simulink model "sst_cllc_ttype_inv"  (R2026a)
settings: Solver=ode23tb  StopTime=simlength  FixedStep=tc  MaxStep=glb_time.tc
values from neighbouring files (symbols this model uses):
  afe_ctrl = ctrl_afe_setup(glb_time.ts_afe, grid_emu.omega_grid_nom)    [init_model.m]
  cllc_ctrl = ctrl_cllc_setup(kp_udc, ki_udc, kp_idc, ki_idc)    [init_model.m]
  glb_time = timing_setup(fpwm_afe, trgo_afe, fpwm_inv, trgo_inv, fpwm_single_phase_inv, trgo_single_phase_inv, fpwm_dab, trgo_dab,      fpwm_psfbc, trgo_psfbc, fpwm_isop_rail, trgo_isop_rail, fpwm_cllc, trgo_cllc, t_measure, tc_factor, tc_decimation, delay_pwm, dead_time_afe,      dead_time_inv, dead_time_single_phase_inv, dead_time_dab, dead_time_psfbc, dead_time_isop_rail, dead_time_cllc)    [init_model.m]
  grid_emu = grid_three_phase_emulator('Dyn11', delta_star, grid_nominal_power, application_voltage, us1, us2, fgrid,                  eq_grid_inductance, eq_grid_resistance, eta, ucc, i1m, p_iron, n1, n2, core_area, core_length, mur,                  up_xi_pu_ref, up_eta_pu_ref, un_xi_pu_ref, un_eta_pu_ref)    [init_model.m]
  lithium_ion_battery_1 = lithium_ion_battery_setup(nominal_battery_voltage_1, nominal_battery_power, initial_battery_soc, glb_time.ts_dab)    [init_model.m]
  omega_set = frequency_set*2*pi    (= 1884.95559215)    [init_model.m]
  single_phase_inverter_ctrl = ctrl_single_phase_inverter_setup(glb_time.ts_inv, pres_ctrl.omega_set,      dqvector_pi.kp_inv, dqvector_pi.ki_inv, pres_ctrl.kp_rpi, pres_ctrl.ki_rpi, pres_ctrl.delta_rpi)    [init_model.m]
  sst_num_of_modules = 2    [init_model.m]
undefined symbols (not defined in the file or in its folder): hwdata
libraries: fl_lib x62, nesl_utility x38, discrete_time_low_pass_filter x8, full_bridge_ideal_switch x4, full_bridge_mosfet_based_with_thermal_model x4, full_bridge_mosfet_based_with_thermal_model_zvs x4, lithium_ion_battery x2, single_phase_transformer x2, dab_single_phase_pwm_modulator x2, dclink_for_three_levels x2, full_bridge_three_level_ttype_ideal_switch_based_model x2, full_bridge_three_level_ttype_mosfet_based_model x2
(part 4 of 5)

== system sst_cllc_ttype_inv/single_phase_inverter_modA/single phase inverter control/single_phase_inverter_ctrl/scopes ==
  Bus Creator1 : BusCreator  Inputs=3
  Bus Creator2 : BusCreator  Inputs=2
  Bus Creator3 : BusCreator  Inputs=2
  Bus Creator4 : BusCreator  Inputs=2
  single phase inverter tracking current scope 1 : Scope  NumInputPorts=2
      settings: ActiveDisplayYMinimum=-1.23468017578125  ActiveDisplayYMaximum=1.23419189453125  DataLoggingVariableName=ScopeData12
  single phase inverter tracking current scope 2 : Scope  NumInputPorts=2
      settings: ActiveDisplayYMinimum=-1.2603759765625  ActiveDisplayYMaximum=1.2652587890625  DataLoggingVariableName=ScopeData2
  wires:
  Bus Creator1/1 -> single phase inverter tracking current scope 1/2  "is_tracking"
  [i_out_alphabeta_ref] -> Bus Creator1/2  "i_out_inverter_pu_ref"
  [afe_current_output_pu] -> Bus Creator1/3  "inverter_current_output_pu"
  [afe_voltage_output_pu] -> Bus Creator2/1  "inverter_voltage_output_pu"
  Bus Creator2/1 -> single phase inverter tracking current scope 1/1  "load"
  [inverter_current_output_pu_reference] -> Bus Creator1/1  "inverter_current_output_pu_reference"
  [afe_current_output_pu] -> Bus Creator2/2  "inverter_current_output_pu"
  [u_ctrl_out] -> Bus Creator3/1  "u_ctrl_out"
  [afe_voltage_output_pu] -> Bus Creator3/2  "inverter_voltage_output_pu"
  Bus Creator3/1 -> single phase inverter tracking current scope 2/2  "u_load"
  [afe_current_output_pu] -> Bus Creator4/2  "inverter_current_output_pu"
  [i_out_alphabeta_ref] -> Bus Creator4/1  "i_out_alphabeta_ref"
  Bus Creator4/1 -> single phase inverter tracking current scope 2/1  "i_load"

== system sst_cllc_ttype_inv/single_phase_inverter_modA/single phase inverter control/single_phase_inverter_ctrl/single_phase_current_control ==
  inverter_current_output_pu_reference : Inport
  current_reference_generation : Subsystem
  dqpi_current_controller : Subsystem
  u_ctrl_out : Outport
  tag scope: i_out_alphabeta_ref=scoped, inverter_current_output_pu_reference=scoped, u_ctrl_out=scoped
  wires:
  current_reference_generation/1(is_ref) -> [i_out_alphabeta_ref]  "i_out_inverter_pu_ref"
  dqpi_current_controller/1(u_out) -> u_ctrl_out/1, [u_ctrl_out]  "u_ctrl_out"
  [phase_grid] -> current_reference_generation/2(phase)
  inverter_current_output_pu_reference/1 -> current_reference_generation/1(mag_ref), [inverter_current_output_pu_reference]
  current_reference_generation/2(id_ref) -> dqpi_current_controller/1(id_ref)

== system sst_cllc_ttype_inv/single_phase_inverter_modA/single phase inverter control/single_phase_inverter_ctrl/single_phase_pll ==
  input : Inport
  Constant : Constant
  Constant2 : Constant  Value=0
  Scope : Scope  NumInputPorts=2
      settings: ActiveDisplayYMinimum=-3.2854912154015015  ActiveDisplayYMaximum=3.4773424919151528
  Sum : Sum  Inputs=|++
  Sum1 : Sum  Inputs=|++
  Terminator : Terminator
  Terminator1 : Terminator
  Terminator2 : Terminator
  Unit Delay1 : UnitDelay  SampleTime=-1
  alphabeta2xieta : MATLAB Function  TreatAsAtomicUnit=on
  bounder2 : MATLAB Function  TreatAsAtomicUnit=on
  double_integrator_observer : Subsystem
  freq_pll : Gain  Gain=1/2/pi
  omega_int_ts : Gain  Gain=omega_set * glb_time.ts_inv
  pi-ctrl : Subsystem  mask{kp=1, ki=0, ts=glb_time.ts_inv, sat_pos=2, sat_neg=-2}
  ualpha_pll : Gain
  ubeta_pll : Gain
  ueta_pll : Gain  Gain=-1
  ueta_pll_flt : discrete_time_low_pass_filter/discrete-time-low-pass-filter  tau=2/omega_set  ts=glb_time.ts_inv
  uxi_pll : Gain
  uxi_pll_flt : discrete_time_low_pass_filter/discrete-time-low-pass-filter  tau=2/omega_set  ts=glb_time.ts_inv
  xieta2alphabeta : MATLAB Function  TreatAsAtomicUnit=on
  phase_pll_hat : Outport
  omega_pll_hat : Outport  Port=2
  wires:
  Sum/1 -> bounder2/1(u)
  alphabeta2xieta/1(xi) -> uxi_pll/1, uxi_pll_flt/1
  xieta2alphabeta/2(beta) -> ubeta_pll/1
  alphabeta2xieta/2(eta) -> ueta_pll/1, ueta_pll_flt/1
  omega_int_ts/1 -> freq_pll/1, Sum/1
  double_integrator_observer/1(phase_hat) -> Scope/1, phase_pll_hat/1  "phase_pll_hat"
  input/1 -> alphabeta2xieta/1(alpha)
  freq_pll/1 -> Terminator1/1  "freq_pll"
  ueta_pll_flt/1 -> xieta2alphabeta/2(eta)
  uxi_pll_flt/1 -> xieta2alphabeta/1(xi)
  ueta_pll/1 -> pi-ctrl/1(x)
  Sum1/1 -> omega_int_ts/1  "freq_pll"
  Constant2/1 -> pi-ctrl/2(xref)
  uxi_pll/1 -> Terminator2/1
  ubeta_pll/1 -> alphabeta2xieta/2(beta)
  xieta2alphabeta/1(alpha) -> ualpha_pll/1
  pi-ctrl/1(u) -> Sum1/1
  Constant/1 -> Sum1/2
  Unit Delay1/1 -> Sum/2, alphabeta2xieta/3(gamma), xieta2alphabeta/3(gamma), double_integrator_observer/1(theta)
  bounder2/1(y) -> Unit Delay1/1  "theta_hat_bounded"
  double_integrator_observer/2(omega_hat) -> Scope/2, omega_pll_hat/1  "omega_pll_hat"
  ualpha_pll/1 -> Terminator/1

== system sst_cllc_ttype_inv/single_phase_inverter_modA/single phase inverter control/single_phase_inverter_ctrl/storage_data ==
  To Workspace : ToWorkspace  VariableName=inverter_voltage_output_pu_sim  SampleTime=-1
      settings: MaxDataPoints=glb_time.Ns_inv  Save2DSignal=2-D array (concatenate along first dimension)
  To Workspace1 : ToWorkspace  VariableName=inverter_current_output_pu_sim  SampleTime=-1
      settings: MaxDataPoints=glb_time.Ns_inv  Save2DSignal=2-D array (concatenate along first dimension)
  To Workspace10 : ToWorkspace  VariableName=iq_pu_ref_sim  SampleTime=-1
      settings: MaxDataPoints=glb_time.Ns_inv  Save2DSignal=2-D array (concatenate along first dimension)
  To Workspace11 : ToWorkspace  VariableName=iq_pu_sim  SampleTime=-1
      settings: MaxDataPoints=glb_time.Ns_inv  Save2DSignal=2-D array (concatenate along first dimension)
  To Workspace12 : ToWorkspace  VariableName=ud_ctrl_out_sim  SampleTime=-1
      settings: MaxDataPoints=glb_time.Ns_inv  Save2DSignal=2-D array (concatenate along first dimension)
  To Workspace13 : ToWorkspace  VariableName=uq_ctrl_out_sim  SampleTime=-1
      settings: MaxDataPoints=glb_time.Ns_inv  Save2DSignal=2-D array (concatenate along first dimension)
  To Workspace2 : ToWorkspace  VariableName=inverter_current_output_pu_reference_sim  SampleTime=-1
      settings: MaxDataPoints=glb_time.Ns_inv  Save2DSignal=2-D array (concatenate along first dimension)
  To Workspace3 : ToWorkspace  VariableName=i_out_inverter_pu_ref_sim  SampleTime=-1
      settings: MaxDataPoints=glb_time.Ns_inv  Save2DSignal=2-D array (concatenate along first dimension)
  To Workspace4 : ToWorkspace  VariableName=u_ctrl_out_sim  SampleTime=-1
      settings: MaxDataPoints=glb_time.Ns_inv  Save2DSignal=2-D array (concatenate along first dimension)
  To Workspace5 : ToWorkspace  VariableName=time_ts_inv_sim  SampleTime=-1
      settings: MaxDataPoints=glb_time.Ns_inv  Save2DSignal=2-D array (concatenate along first dimension)
  To Workspace6 : ToWorkspace  VariableName=i_alpha_pu_sim  SampleTime=-1
      settings: MaxDataPoints=glb_time.Ns_inv  Save2DSignal=2-D array (concatenate along first dimension)
  To Workspace7 : ToWorkspace  VariableName=i_beta_pu_sim  SampleTime=-1
      settings: MaxDataPoints=glb_time.Ns_inv  Save2DSignal=2-D array (concatenate along first dimension)
  To Workspace8 : ToWorkspace  VariableName=id_pu_ref_sim  SampleTime=-1
      settings: MaxDataPoints=glb_time.Ns_inv  Save2DSignal=2-D array (concatenate along first dimension)
  To Workspace9 : ToWorkspace  VariableName=id_pu_sim  SampleTime=-1
      settings: MaxDataPoints=glb_time.Ns_inv  Save2DSignal=2-D array (concatenate along first dimension)
  wires:
  [afe_voltage_output_pu] -> To Workspace/1  "inverter_voltage_output_pu"
  [afe_current_output_pu] -> To Workspace1/1  "inverter_current_output_pu"
  [inverter_current_output_pu_reference] -> To Workspace2/1  "inverter_current_output_pu_reference"
  [i_out_alphabeta_ref] -> To Workspace3/1  "i_out_inverter_pu_ref"
  [u_ctrl_out] -> To Workspace4/1  "u_ctrl_out"
  [local_time] -> To Workspace5/1
  [i_alpha] -> To Workspace6/1
  [i_beta] -> To Workspace7/1
  [id_ref] -> To Workspace8/1
  [id] -> To Workspace9/1
  [iq_ref] -> To Workspace10/1
  [iq] -> To Workspace11/1
  [ud_ctrl] -> To Workspace12/1
  [uq_ctrl] -> To Workspace13/1

== system sst_cllc_ttype_inv/single_phase_inverter_modB/single phase inverter control/single_phase_inverter_ctrl/scopes ==
  Bus Creator1 : BusCreator  Inputs=3
  Bus Creator2 : BusCreator  Inputs=2
  Bus Creator3 : BusCreator  Inputs=2
  Bus Creator4 : BusCreator  Inputs=2
  single phase inverter tracking current scope 1 : Scope  NumInputPorts=2
      settings: ActiveDisplayYMinimum=-1.23468017578125  ActiveDisplayYMaximum=1.23419189453125  DataLoggingVariableName=ScopeData12
  single phase inverter tracking current scope 2 : Scope  NumInputPorts=2
      settings: ActiveDisplayYMinimum=-1.2603759765625  ActiveDisplayYMaximum=1.2652587890625  DataLoggingVariableName=ScopeData2
  wires:
  Bus Creator4/1 -> single phase inverter tracking current scope 2/1  "i_load"
  [i_out_alphabeta_ref] -> Bus Creator4/1  "i_out_alphabeta_ref"
  [afe_current_output_pu] -> Bus Creator4/2  "inverter_current_output_pu"
  Bus Creator3/1 -> single phase inverter tracking current scope 2/2  "u_load"
  [afe_voltage_output_pu] -> Bus Creator3/2  "inverter_voltage_output_pu"
  [u_ctrl_out] -> Bus Creator3/1  "u_ctrl_out"
  [afe_current_output_pu] -> Bus Creator2/2  "inverter_current_output_pu"
  [inverter_current_output_pu_reference] -> Bus Creator1/1  "inverter_current_output_pu_reference"
  Bus Creator2/1 -> single phase inverter tracking current scope 1/1  "load"
  [afe_voltage_output_pu] -> Bus Creator2/1  "inverter_voltage_output_pu"
  [afe_current_output_pu] -> Bus Creator1/3  "inverter_current_output_pu"
  [i_out_alphabeta_ref] -> Bus Creator1/2  "i_out_inverter_pu_ref"
  Bus Creator1/1 -> single phase inverter tracking current scope 1/2  "is_tracking"

== system sst_cllc_ttype_inv/single_phase_inverter_modB/single phase inverter control/single_phase_inverter_ctrl/single_phase_current_control ==
  inverter_current_output_pu_reference : Inport
  current_reference_generation : Subsystem
  dqpi_current_controller : Subsystem
  u_ctrl_out : Outport
  tag scope: i_out_alphabeta_ref=scoped, inverter_current_output_pu_reference=scoped, u_ctrl_out=scoped
  wires:
  current_reference_generation/2(id_ref) -> dqpi_current_controller/1(id_ref)
  inverter_current_output_pu_reference/1 -> [inverter_current_output_pu_reference], current_reference_generation/1(mag_ref)
  [phase_grid] -> current_reference_generation/2(phase)
  dqpi_current_controller/1(u_out) -> [u_ctrl_out], u_ctrl_out/1  "u_ctrl_out"
  current_reference_generation/1(is_ref) -> [i_out_alphabeta_ref]  "i_out_inverter_pu_ref"

== system sst_cllc_ttype_inv/single_phase_inverter_modB/single phase inverter control/single_phase_inverter_ctrl/single_phase_pll ==
  input : Inport
  Constant : Constant
  Constant2 : Constant  Value=0
  Scope : Scope  NumInputPorts=2
      settings: ActiveDisplayYMinimum=-3.2854912154015015  ActiveDisplayYMaximum=3.4773424919151528
  Sum : Sum  Inputs=|++
  Sum1 : Sum  Inputs=|++
  Terminator : Terminator
  Terminator1 : Terminator
  Terminator2 : Terminator
  Unit Delay1 : UnitDelay  SampleTime=-1
  alphabeta2xieta : MATLAB Function  TreatAsAtomicUnit=on
  bounder2 : MATLAB Function  TreatAsAtomicUnit=on
  double_integrator_observer : Subsystem
  freq_pll : Gain  Gain=1/2/pi
  omega_int_ts : Gain  Gain=omega_set * glb_time.ts_inv
  pi-ctrl : Subsystem  mask{kp=1, ki=0, ts=glb_time.ts_inv, sat_pos=2, sat_neg=-2}
  ualpha_pll : Gain
  ubeta_pll : Gain
  ueta_pll : Gain  Gain=-1
  ueta_pll_flt : discrete_time_low_pass_filter/discrete-time-low-pass-filter  tau=2/omega_set  ts=glb_time.ts_inv
  uxi_pll : Gain
  uxi_pll_flt : discrete_time_low_pass_filter/discrete-time-low-pass-filter  tau=2/omega_set  ts=glb_time.ts_inv
  xieta2alphabeta : MATLAB Function  TreatAsAtomicUnit=on
  phase_pll_hat : Outport
  omega_pll_hat : Outport  Port=2
  wires:
  ualpha_pll/1 -> Terminator/1
  double_integrator_observer/2(omega_hat) -> omega_pll_hat/1, Scope/2  "omega_pll_hat"
  bounder2/1(y) -> Unit Delay1/1  "theta_hat_bounded"
  Unit Delay1/1 -> double_integrator_observer/1(theta), xieta2alphabeta/3(gamma), alphabeta2xieta/3(gamma), Sum/2
  Constant/1 -> Sum1/2
  pi-ctrl/1(u) -> Sum1/1
  xieta2alphabeta/1(alpha) -> ualpha_pll/1
  ubeta_pll/1 -> alphabeta2xieta/2(beta)
  uxi_pll/1 -> Terminator2/1
  Constant2/1 -> pi-ctrl/2(xref)
  Sum1/1 -> omega_int_ts/1  "freq_pll"
  ueta_pll/1 -> pi-ctrl/1(x)
  uxi_pll_flt/1 -> xieta2alphabeta/1(xi)
  ueta_pll_flt/1 -> xieta2alphabeta/2(eta)
  freq_pll/1 -> Terminator1/1  "freq_pll"
  input/1 -> alphabeta2xieta/1(alpha)
  double_integrator_observer/1(phase_hat) -> phase_pll_hat/1, Scope/1  "phase_pll_hat"
  omega_int_ts/1 -> Sum/1, freq_pll/1
  alphabeta2xieta/2(eta) -> ueta_pll_flt/1, ueta_pll/1
  xieta2alphabeta/2(beta) -> ubeta_pll/1
  alphabeta2xieta/1(xi) -> uxi_pll_flt/1, uxi_pll/1
  Sum/1 -> bounder2/1(u)

== system sst_cllc_ttype_inv/single_phase_inverter_modB/single phase inverter control/single_phase_inverter_ctrl/storage_data ==
  To Workspace : ToWorkspace  VariableName=inverter_voltage_output_pu_sim  SampleTime=-1
      settings: MaxDataPoints=glb_time.Ns_inv  Save2DSignal=2-D array (concatenate along first dimension)
  To Workspace1 : ToWorkspace  VariableName=inverter_current_output_pu_sim  SampleTime=-1
      settings: MaxDataPoints=glb_time.Ns_inv  Save2DSignal=2-D array (concatenate along first dimension)
  To Workspace10 : ToWorkspace  VariableName=iq_pu_ref_sim  SampleTime=-1
      settings: MaxDataPoints=glb_time.Ns_inv  Save2DSignal=2-D array (concatenate along first dimension)
  To Workspace11 : ToWorkspace  VariableName=iq_pu_sim  SampleTime=-1
      settings: MaxDataPoints=glb_time.Ns_inv  Save2DSignal=2-D array (concatenate along first dimension)
  To Workspace12 : ToWorkspace  VariableName=ud_ctrl_out_sim  SampleTime=-1
      settings: MaxDataPoints=glb_time.Ns_inv  Save2DSignal=2-D array (concatenate along first dimension)
  To Workspace13 : ToWorkspace  VariableName=uq_ctrl_out_sim  SampleTime=-1
      settings: MaxDataPoints=glb_time.Ns_inv  Save2DSignal=2-D array (concatenate along first dimension)
  To Workspace2 : ToWorkspace  VariableName=inverter_current_output_pu_reference_sim  SampleTime=-1
      settings: MaxDataPoints=glb_time.Ns_inv  Save2DSignal=2-D array (concatenate along first dimension)
  To Workspace3 : ToWorkspace  VariableName=i_out_inverter_pu_ref_sim  SampleTime=-1
      settings: MaxDataPoints=glb_time.Ns_inv  Save2DSignal=2-D array (concatenate along first dimension)
  To Workspace4 : ToWorkspace  VariableName=u_ctrl_out_sim  SampleTime=-1
      settings: MaxDataPoints=glb_time.Ns_inv  Save2DSignal=2-D array (concatenate along first dimension)
  To Workspace5 : ToWorkspace  VariableName=time_ts_inv_sim  SampleTime=-1
      settings: MaxDataPoints=glb_time.Ns_inv  Save2DSignal=2-D array (concatenate along first dimension)
  To Workspace6 : ToWorkspace  VariableName=i_alpha_pu_sim  SampleTime=-1
      settings: MaxDataPoints=glb_time.Ns_inv  Save2DSignal=2-D array (concatenate along first dimension)
  To Workspace7 : ToWorkspace  VariableName=i_beta_pu_sim  SampleTime=-1
      settings: MaxDataPoints=glb_time.Ns_inv  Save2DSignal=2-D array (concatenate along first dimension)
  To Workspace8 : ToWorkspace  VariableName=id_pu_ref_sim  SampleTime=-1
      settings: MaxDataPoints=glb_time.Ns_inv  Save2DSignal=2-D array (concatenate along first dimension)
  To Workspace9 : ToWorkspace  VariableName=id_pu_sim  SampleTime=-1
      settings: MaxDataPoints=glb_time.Ns_inv  Save2DSignal=2-D array (concatenate along first dimension)
  wires:
  [uq_ctrl] -> To Workspace13/1
  [ud_ctrl] -> To Workspace12/1
  [iq] -> To Workspace11/1
  [iq_ref] -> To Workspace10/1
  [id] -> To Workspace9/1
  [id_ref] -> To Workspace8/1
  [i_beta] -> To Workspace7/1
  [i_alpha] -> To Workspace6/1
  [local_time] -> To Workspace5/1
  [u_ctrl_out] -> To Workspace4/1  "u_ctrl_out"
  [i_out_alphabeta_ref] -> To Workspace3/1  "i_out_inverter_pu_ref"
  [inverter_current_output_pu_reference] -> To Workspace2/1  "inverter_current_output_pu_reference"
  [afe_current_output_pu] -> To Workspace1/1  "inverter_current_output_pu"
  [afe_voltage_output_pu] -> To Workspace/1  "inverter_voltage_output_pu"

== system sst_cllc_ttype_inv/dcdc_cllc_modA/dcdc_with_galvanic_isolation/full-bridge_1/full-bridge_ideal_switch_based/data_measure ==
  m : Inport
  Bus Selector1 : BusSelector  OutputSignals=ideal_switch_current_Q2,ideal_switch_voltage_Q2
  Bus Selector2 : BusSelector  OutputSignals=ideal_switch_current_Q1,ideal_switch_voltage_Q1
  tag scope: idevice_ids_cllc_Q1_modA=global, idevice_ids_cllc_Q2_modA=global, idevice_uds_cllc_Q1_modA=global, idevice_uds_cllc_Q2_modA=global
  wires:
  Bus Selector1/1 -> [idevice_ids_cllc_Q2_modA]  "<ideal_switch_current_Q2>"
  Bus Selector1/2 -> [idevice_uds_cllc_Q2_modA]  "<ideal_switch_voltage_Q2>"
  m/1 -> Bus Selector2/1, Bus Selector1/1
  Bus Selector2/1 -> [idevice_ids_cllc_Q1_modA]  "<ideal_switch_current_Q1>"
  Bus Selector2/2 -> [idevice_uds_cllc_Q1_modA]  "<ideal_switch_voltage_Q1>"

== system sst_cllc_ttype_inv/dcdc_cllc_modA/dcdc_with_galvanic_isolation/full-bridge_1/full-bridge_mosfet_based_with_thermal_model/data_measure ==
  m : Inport
  tag scope: inverter_1_cllc_mosfet_modA=global
  wires:
  m/1 -> [inverter_1_cllc_mosfet_modA]

== system sst_cllc_ttype_inv/dcdc_cllc_modA/dcdc_with_galvanic_isolation/full-bridge_1/full-bridge_mosfet_based_with_thermal_model_zvs/data_measure ==
  m : Inport
  tag scope: inverter_1_cllc_mosfet_zvs_modA=global
  wires:
  m/1 -> [inverter_1_cllc_mosfet_zvs_modA]

== system sst_cllc_ttype_inv/dcdc_cllc_modA/dcdc_with_galvanic_isolation/full-bridge_2/full-bridge_ideal_switch_based/data_measure ==
  m : Inport
  Bus Selector1 : BusSelector  OutputSignals=ideal_switch_current_Q2,ideal_switch_voltage_Q2
  Bus Selector2 : BusSelector  OutputSignals=ideal_switch_current_Q1,ideal_switch_voltage_Q1
  tag scope: idevice_ids_cllc_Q5_modA=global, idevice_ids_cllc_Q6_modA=global, idevice_uds_cllc_Q5_modA=global, idevice_uds_cllc_Q6_modA=global
  wires:
  Bus Selector1/1 -> [idevice_ids_cllc_Q6_modA]  "<ideal_switch_current_Q2>"
  Bus Selector1/2 -> [idevice_uds_cllc_Q6_modA]  "<ideal_switch_voltage_Q2>"
  m/1 -> Bus Selector2/1, Bus Selector1/1
  Bus Selector2/1 -> [idevice_ids_cllc_Q5_modA]  "<ideal_switch_current_Q1>"
  Bus Selector2/2 -> [idevice_uds_cllc_Q5_modA]  "<ideal_switch_voltage_Q1>"

== system sst_cllc_ttype_inv/dcdc_cllc_modA/dcdc_with_galvanic_isolation/full-bridge_2/full-bridge_mosfet_based_with_thermal_model/data_measure ==
  m : Inport
  tag scope: inverter_2_cllc_mosfet_modA=global
  wires:
  m/1 -> [inverter_2_cllc_mosfet_modA]

== system sst_cllc_ttype_inv/dcdc_cllc_modA/dcdc_with_galvanic_isolation/full-bridge_2/full-bridge_mosfet_based_with_thermal_model_zvs/data_measure ==
  m : Inport
  tag scope: inverter_2_cllc_mosfet_zvs_modA=global
  wires:
  m/1 -> [inverter_2_cllc_mosfet_zvs_modA]

== system sst_cllc_ttype_inv/dcdc_cllc_modA/input_current_control/input_current_control/inner_ctrl/current_control ==
  i_ref : Inport
  i : Inport  Port=2
  Gain : Gain  Gain=-1
  Sum2 : Sum  Inputs=+-  OutDataTypeStr=double  AccumDataTypeStr=double  SaturateOnIntegerOverflow=on
  Unit Delay2 : UnitDelay  SampleTime=-1
  i_ctrl : Subsystem
  ctrli_out : Outport
  wires:
  i/1 -> Sum2/2
  i_ref/1 -> Sum2/1
  Sum2/1 -> i_ctrl/1(i_tilde)
  Gain/1 -> Unit Delay2/1
  i_ctrl/1(phase_shift) -> Gain/1
  Unit Delay2/1 -> ctrli_out/1  "current_ctrl_output"

== system sst_cllc_ttype_inv/dcdc_cllc_modA/input_current_control/input_current_control/outer_ctrl/current_control ==
  iout_ref : Inport
  iout : Inport  Port=2
  Gain : Gain
  Sum2 : Sum  Inputs=+-  OutDataTypeStr=double  AccumDataTypeStr=double  SaturateOnIntegerOverflow=on
  Unit Delay2 : UnitDelay  SampleTime=-1
  iout_ctrl : Subsystem
  ctrli_out : Outport
  wires:
  Unit Delay2/1 -> ctrli_out/1  "current_ctrl_output"
  iout_ctrl/1(phase_shift) -> Gain/1
  Gain/1 -> Unit Delay2/1
  Sum2/1 -> iout_ctrl/1(i_tilde)
  iout_ref/1 -> Sum2/1
  iout/1 -> Sum2/2

== system sst_cllc_ttype_inv/dcdc_cllc_modB/dcdc_with_galvanic_isolation/full-bridge_1/full-bridge_ideal_switch_based/data_measure ==
  m : Inport
  Bus Selector1 : BusSelector  OutputSignals=ideal_switch_current_Q2,ideal_switch_voltage_Q2
  Bus Selector2 : BusSelector  OutputSignals=ideal_switch_current_Q1,ideal_switch_voltage_Q1
  tag scope: idevice_ids_cllc_Q1_modB=global, idevice_ids_cllc_Q2_modB=global, idevice_uds_cllc_Q1_modB=global, idevice_uds_cllc_Q2_modB=global
  wires:
  Bus Selector2/2 -> [idevice_uds_cllc_Q1_modB]  "<ideal_switch_voltage_Q1>"
  Bus Selector2/1 -> [idevice_ids_cllc_Q1_modB]  "<ideal_switch_current_Q1>"
  m/1 -> Bus Selector1/1, Bus Selector2/1
  Bus Selector1/2 -> [idevice_uds_cllc_Q2_modB]  "<ideal_switch_voltage_Q2>"
  Bus Selector1/1 -> [idevice_ids_cllc_Q2_modB]  "<ideal_switch_current_Q2>"

== system sst_cllc_ttype_inv/dcdc_cllc_modB/dcdc_with_galvanic_isolation/full-bridge_1/full-bridge_mosfet_based_with_thermal_model/data_measure ==
  m : Inport
  tag scope: inverter_1_cllc_mosfet_modB=global
  wires:
  m/1 -> [inverter_1_cllc_mosfet_modB]

== system sst_cllc_ttype_inv/dcdc_cllc_modB/dcdc_with_galvanic_isolation/full-bridge_1/full-bridge_mosfet_based_with_thermal_model_zvs/data_measure ==
  m : Inport
  tag scope: inverter_1_cllc_mosfet_zvs_modB=global
  wires:
  m/1 -> [inverter_1_cllc_mosfet_zvs_modB]

== system sst_cllc_ttype_inv/dcdc_cllc_modB/dcdc_with_galvanic_isolation/full-bridge_2/full-bridge_ideal_switch_based/data_measure ==
  m : Inport
  Bus Selector1 : BusSelector  OutputSignals=ideal_switch_current_Q2,ideal_switch_voltage_Q2
  Bus Selector2 : BusSelector  OutputSignals=ideal_switch_current_Q1,ideal_switch_voltage_Q1
  tag scope: idevice_ids_cllc_Q5_modB=global, idevice_ids_cllc_Q6_modB=global, idevice_uds_cllc_Q5_modB=global, idevice_uds_cllc_Q6_modB=global
  wires:
  Bus Selector2/2 -> [idevice_uds_cllc_Q5_modB]  "<ideal_switch_voltage_Q1>"
  Bus Selector2/1 -> [idevice_ids_cllc_Q5_modB]  "<ideal_switch_current_Q1>"
  m/1 -> Bus Selector1/1, Bus Selector2/1
  Bus Selector1/2 -> [idevice_uds_cllc_Q6_modB]  "<ideal_switch_voltage_Q2>"
  Bus Selector1/1 -> [idevice_ids_cllc_Q6_modB]  "<ideal_switch_current_Q2>"

== system sst_cllc_ttype_inv/dcdc_cllc_modB/dcdc_with_galvanic_isolation/full-bridge_2/full-bridge_mosfet_based_with_thermal_model/data_measure ==
  m : Inport
  Bus Selector : BusSelector  OutputSignals=mosfet_ploss_Q1,mosfet_voltage_Q1,mosfet_current_Q1,mosfet_JH_temp_Q1,mosfet_HA_temp_Q1
  Bus Selector1 : BusSelector  OutputSignals=mosfet_ploss_Q2,mosfet_voltage_Q2,mosfet_current_Q2,mosfet_JH_temp_Q2,mosfet_HA_temp_Q2
  tag scope: inverter_2_cllc_mosfet_modA=global, mosfet_HA_temp_cllc_Q5=global, mosfet_HA_temp_cllc_Q6=global, mosfet_JH_temp_cllc_Q5=global, mosfet_JH_temp_cllc_Q6=global, mosfet_ids_cllc_Q5=global, mosfet_ids_cllc_Q6=global, mosfet_plosses_cllc_Q5=global, mosfet_plosses_cllc_Q6=global, mosfet_uds_cllc_Q5=global, mosfet_uds_cllc_Q6=global
  wires:
  m/1 -> [inverter_2_cllc_mosfet_modA], Bus Selector1/1, Bus Selector/1
  Bus Selector1/1 -> [mosfet_plosses_cllc_Q6]  "<mosfet_ploss_Q2>"
  Bus Selector/2 -> [mosfet_uds_cllc_Q5]  "<mosfet_voltage_Q1>"
  Bus Selector/3 -> [mosfet_ids_cllc_Q5]  "<mosfet_current_Q1>"
  Bus Selector1/4 -> [mosfet_JH_temp_cllc_Q6]  "<mosfet_JH_temp_Q2>"
  Bus Selector/5 -> [mosfet_HA_temp_cllc_Q5]  "<mosfet_HA_temp_Q1>"
  Bus Selector/4 -> [mosfet_JH_temp_cllc_Q5]  "<mosfet_JH_temp_Q1>"
  Bus Selector1/5 -> [mosfet_HA_temp_cllc_Q6]  "<mosfet_HA_temp_Q2>"
  Bus Selector1/2 -> [mosfet_uds_cllc_Q6]  "<mosfet_voltage_Q2>"
  Bus Selector1/3 -> [mosfet_ids_cllc_Q6]  "<mosfet_current_Q2>"
  Bus Selector/1 -> [mosfet_plosses_cllc_Q5]  "<mosfet_ploss_Q1>"

== system sst_cllc_ttype_inv/dcdc_cllc_modB/dcdc_with_galvanic_isolation/full-bridge_2/full-bridge_mosfet_based_with_thermal_model_zvs/data_measure ==
  m : Inport
  tag scope: inverter_2_cllc_mosfet_zvs_modB=global
  wires:
  m/1 -> [inverter_2_cllc_mosfet_zvs_modB]

== system sst_cllc_ttype_inv/dcdc_cllc_modB/input_current_control/input_current_control/inner_ctrl/current_control ==
  i_ref : Inport
  i : Inport  Port=2
  Gain : Gain  Gain=-1
  Sum2 : Sum  Inputs=+-  OutDataTypeStr=double  AccumDataTypeStr=double  SaturateOnIntegerOverflow=on
  Unit Delay2 : UnitDelay  SampleTime=-1
  i_ctrl : Subsystem
  ctrli_out : Outport
  wires:
  Unit Delay2/1 -> ctrli_out/1  "current_ctrl_output"
  i_ctrl/1(phase_shift) -> Gain/1
  Gain/1 -> Unit Delay2/1
  Sum2/1 -> i_ctrl/1(i_tilde)
  i_ref/1 -> Sum2/1
  i/1 -> Sum2/2

== system sst_cllc_ttype_inv/dcdc_cllc_modB/input_current_control/input_current_control/outer_ctrl/current_control ==
  iout_ref : Inport
  iout : Inport  Port=2
  Gain : Gain
  Sum2 : Sum  Inputs=+-  OutDataTypeStr=double  AccumDataTypeStr=double  SaturateOnIntegerOverflow=on
  Unit Delay2 : UnitDelay  SampleTime=-1
  iout_ctrl : Subsystem
  ctrli_out : Outport
  wires:
  iout/1 -> Sum2/2
  iout_ref/1 -> Sum2/1
  Sum2/1 -> iout_ctrl/1(i_tilde)
  Gain/1 -> Unit Delay2/1
  iout_ctrl/1(phase_shift) -> Gain/1
  Unit Delay2/1 -> ctrli_out/1  "current_ctrl_output"

== system sst_cllc_ttype_inv/single_phase_inverter_modA/single phase inverter control/single_phase_inverter_ctrl/single_phase_current_control/current_reference_generation ==
  mag_ref : Inport
  phase : Inport  Port=2
  Bus Creator : BusCreator  Inputs=2
  Product : Product
  Product1 : Product
  Sin : Trigonometry  Operator=cos
  Sin1 : Trigonometry
  is_ref : Outport
  id_ref : Outport  Port=2
  wires:
  Sin/1 -> Product/2
  phase/1 -> Sin1/1, Sin/1
  mag_ref/1 -> id_ref/1, Product1/1, Product/1
  Sin1/1 -> Product1/2
  Product/1 -> Bus Creator/1  "is_ref_alpha"
  Product1/1 -> Bus Creator/2  "is_ref_beta"
  Bus Creator/1 -> is_ref/1

== system sst_cllc_ttype_inv/single_phase_inverter_modA/single phase inverter control/single_phase_inverter_ctrl/single_phase_current_control/dqpi_current_controller ==
  id_ref : Inport
  Bus Creator : BusCreator  Inputs=3
  Bus Creator1 : BusCreator  Inputs=3
  alpha_beta currents : Scope  NumInputPorts=3
      settings: ActiveDisplayYMinimum=-43.020049026506776  ActiveDisplayYMaximum=15.212667801061009  DataLoggingVariableName=ScopeData2
  alphabeta2dq : Subsystem
  dq2alphabeta : Subsystem
  dq_vector_pi : Subsystem
  dq_vector_pi_tracking : Scope  NumInputPorts=2
      settings: ActiveDisplayYMinimum=-5.8450231123834442  ActiveDisplayYMaximum=20.947282871449747  DataLoggingVariableName=ScopeData8
  i2alphabeta : Subsystem
  u_out : Outport
  tag scope: i_alpha=scoped, i_beta=scoped, id=scoped, id_ref=scoped, iq=scoped, ud_ctrl=scoped, uq_ctrl=scoped
  wires:
  dq2alphabeta/1(alpha) -> u_out/1
  id_ref/1 -> dq_vector_pi/1(id_ref), Bus Creator/1, [id_ref]
  alphabeta2dq/1("d ") -> Bus Creator/2, [id], dq_vector_pi/2(id)  "id"
  alphabeta2dq/2("q ") -> dq_vector_pi/3(iq), Bus Creator1/2, [iq]  "iq"
  [iq_ref] -> dq_vector_pi/4(iq_ref)
  Bus Creator1/1 -> dq_vector_pi_tracking/2
  Bus Creator/1 -> dq_vector_pi_tracking/1
  [ud_ctrl] -> Bus Creator/3
  [uq_ctrl] -> Bus Creator1/3
  [iq_ref] -> Bus Creator1/1
  [afe_current_output_pu] -> alpha_beta currents/1, i2alphabeta/1(i_alpha)  "i_load"
  i2alphabeta/1(i_alpha_out) -> alpha_beta currents/2, [i_alpha], alphabeta2dq/1(alpha)  "i_alpha"
  i2alphabeta/2(i_beta_out) -> [i_beta], alpha_beta currents/3, alphabeta2dq/2(beta)  "i_beta"
  dq_vector_pi/1(ud_ctrl) -> [ud_ctrl], dq2alphabeta/1(d)
  dq_vector_pi/2(uq_ctrl) -> [uq_ctrl], dq2alphabeta/2(q)

== system sst_cllc_ttype_inv/single_phase_inverter_modA/single phase inverter control/single_phase_inverter_ctrl/single_phase_pll/double_integrator_observer ==
  theta : Inport
  Gain : Gain  Gain=afe_ctrl.di_obs.Ldso  Multiplication=Matrix(K*u)
  Gain1 : Gain  Gain=afe_ctrl.di_obs.Adso  Multiplication=Matrix(K*u)
  Gain2 : Gain  Gain=afe_ctrl.di_obs.Cso  Multiplication=Matrix(K*u)
  Selector : Selector  InputPortWidth=2  IndexOptions=Index vector (dialog)  Indices=2  OutputSizes=1
  Sum : Sum  Inputs=-+|
  Sum1 : Sum  Inputs=|++
  Unit Delay : UnitDelay  SampleTime=-1
  bounder1 : MATLAB Function  TreatAsAtomicUnit=on
  bounder2 : MATLAB Function  TreatAsAtomicUnit=on
  kp3 : Gain  Gain=1/grid_emu.omega_grid_nom  SaturateOnIntegerOverflow=on  OutDataTypeStr=Inherit: Same as input  ParamDataTypeStr=Inherit: Same as input
  phase_hat : Outport
  omega_hat : Outport  Port=2
  wires:
  Gain/1 -> Sum1/1
  Gain2/1 -> bounder2/1(u)  "theta_hat"
  Gain1/1 -> Sum1/2
  Sum1/1 -> Unit Delay/1
  Sum/1 -> bounder1/1(u)  "e"
  Unit Delay/1 -> Selector/1, Gain1/1, Gain2/1
  theta/1 -> Sum/2  "theta"
  bounder1/1(y) -> Gain/1  "e_bounded"
  bounder2/1(y) -> phase_hat/1, Sum/1  "theta_hat_bounded"
  Selector/1 -> kp3/1
  kp3/1 -> omega_hat/1

== system sst_cllc_ttype_inv/single_phase_inverter_modA/single phase inverter control/single_phase_inverter_ctrl/single_phase_pll/pi-ctrl ==
  x : Inport
  xref : Inport  Port=2
  1/Ti : Gain  Gain=kp  SaturateOnIntegerOverflow=on  OutDataTypeStr=Inherit: Same as input  ParamDataTypeStr=Inherit: Same as input
  Saturation : Saturate  UpperLimit=sat_pos  LowerLimit=sat_neg
  Sum1 : Sum  Inputs=+++  SaturateOnIntegerOverflow=on
  Sum2 : Sum  Inputs=-+  SaturateOnIntegerOverflow=on
  Sum3 : Sum  Inputs=-+  SaturateOnIntegerOverflow=on
  Unit Delay4 : UnitDelay  SampleTime=-1
  kp : Gain  Gain=ki*ts  SaturateOnIntegerOverflow=on  OutDataTypeStr=Inherit: Same as input  ParamDataTypeStr=Inherit: Same as input
  u : Outport
  wires:
  Saturation/1 -> Sum3/2, u/1
  Unit Delay4/1 -> Sum1/3
  Sum1/1 -> Saturation/1
  Sum3/1 -> Unit Delay4/1
  1/Ti/1 -> Sum3/1, Sum1/1
  Sum2/1 -> 1/Ti/1, kp/1
  kp/1 -> Sum1/2
  x/1 -> Sum2/1
  xref/1 -> Sum2/2

== system sst_cllc_ttype_inv/single_phase_inverter_modB/single phase inverter control/single_phase_inverter_ctrl/single_phase_current_control/current_reference_generation ==
  mag_ref : Inport
  phase : Inport  Port=2
  Bus Creator : BusCreator  Inputs=2
  Product : Product
  Product1 : Product
  Sin : Trigonometry  Operator=cos
  Sin1 : Trigonometry
  is_ref : Outport
  id_ref : Outport  Port=2
  wires:
  Bus Creator/1 -> is_ref/1
  Product1/1 -> Bus Creator/2  "is_ref_beta"
  Product/1 -> Bus Creator/1  "is_ref_alpha"
  Sin1/1 -> Product1/2
  mag_ref/1 -> Product/1, Product1/1, id_ref/1
  phase/1 -> Sin/1, Sin1/1
  Sin/1 -> Product/2

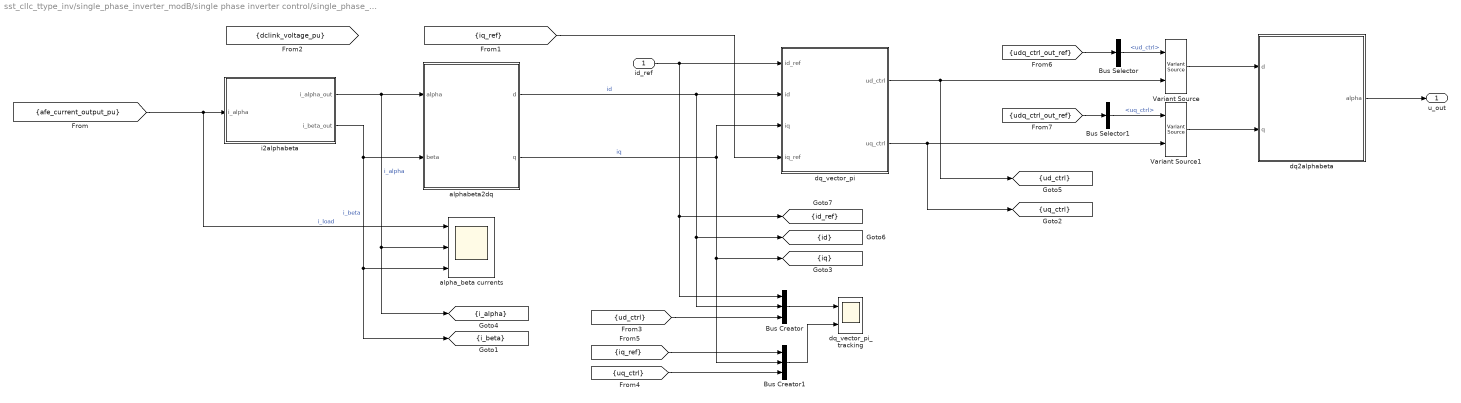
== system sst_cllc_ttype_inv/single_phase_inverter_modB/single phase inverter control/single_phase_inverter_ctrl/single_phase_current_control/dqpi_current_controller ==
  id_ref : Inport
  Bus Creator : BusCreator  Inputs=3
  Bus Creator1 : BusCreator  Inputs=3
  Bus Selector : BusSelector  OutputSignals=ud_ctrl
  Bus Selector1 : BusSelector  OutputSignals=uq_ctrl
  Variant Source : VariantSource  VariantControls={true, false}
  Variant Source1 : VariantSource  VariantControls={true, false}
  alpha_beta currents : Scope  NumInputPorts=3
      settings: ActiveDisplayYMinimum=-43.020049026506776  ActiveDisplayYMaximum=15.212667801061009  DataLoggingVariableName=ScopeData2
  alphabeta2dq : Subsystem
  dq2alphabeta : Subsystem
  dq_vector_pi : Subsystem
  dq_vector_pi_tracking : Scope  NumInputPorts=2
      settings: ActiveDisplayYMinimum=-5.8450231123834442  ActiveDisplayYMaximum=20.947282871449747  DataLoggingVariableName=ScopeData8
  i2alphabeta : Subsystem
  u_out : Outport
  tag scope: i_alpha=scoped, i_beta=scoped, id=scoped, id_ref=scoped, iq=scoped, ud_ctrl=scoped, uq_ctrl=scoped
  wires:
  dq_vector_pi/1(ud_ctrl) -> [ud_ctrl], Variant Source/2
  i2alphabeta/2(i_beta_out) -> alphabeta2dq/2(beta), alpha_beta currents/3, [i_beta]  "i_beta"
  i2alphabeta/1(i_alpha_out) -> alphabeta2dq/1(alpha), [i_alpha], alpha_beta currents/2  "i_alpha"
  [afe_current_output_pu] -> i2alphabeta/1(i_alpha), alpha_beta currents/1  "i_load"
  [iq_ref] -> Bus Creator1/1
  [uq_ctrl] -> Bus Creator1/3
  [ud_ctrl] -> Bus Creator/3
  Bus Creator/1 -> dq_vector_pi_tracking/1
  Bus Creator1/1 -> dq_vector_pi_tracking/2
  [iq_ref] -> dq_vector_pi/4(iq_ref)
  alphabeta2dq/2("q ") -> [iq], Bus Creator1/2, dq_vector_pi/3(iq)  "iq"
  alphabeta2dq/1("d ") -> dq_vector_pi/2(id), [id], Bus Creator/2  "id"
  id_ref/1 -> [id_ref], Bus Creator/1, dq_vector_pi/1(id_ref)
  dq2alphabeta/1(alpha) -> u_out/1
  [udq_ctrl_out_ref] -> Bus Selector/1
  Variant Source/1 -> dq2alphabeta/1(d)
  Bus Selector/1 -> Variant Source/1  "<ud_ctrl>"
  Bus Selector1/1 -> Variant Source1/1  "<uq_ctrl>"
  [udq_ctrl_out_ref] -> Bus Selector1/1
  dq_vector_pi/2(uq_ctrl) -> Variant Source1/2, [uq_ctrl]
  Variant Source1/1 -> dq2alphabeta/2(q)

== system sst_cllc_ttype_inv/single_phase_inverter_modB/single phase inverter control/single_phase_inverter_ctrl/single_phase_pll/double_integrator_observer ==
  theta : Inport
  Gain : Gain  Gain=afe_ctrl.di_obs.Ldso  Multiplication=Matrix(K*u)
  Gain1 : Gain  Gain=afe_ctrl.di_obs.Adso  Multiplication=Matrix(K*u)
  Gain2 : Gain  Gain=afe_ctrl.di_obs.Cso  Multiplication=Matrix(K*u)
  Selector : Selector  InputPortWidth=2  IndexOptions=Index vector (dialog)  Indices=2  OutputSizes=1
  Sum : Sum  Inputs=-+|
  Sum1 : Sum  Inputs=|++
  Unit Delay : UnitDelay  SampleTime=-1
  bounder1 : MATLAB Function  TreatAsAtomicUnit=on
  bounder2 : MATLAB Function  TreatAsAtomicUnit=on
  kp3 : Gain  Gain=1/grid_emu.omega_grid_nom  SaturateOnIntegerOverflow=on  OutDataTypeStr=Inherit: Same as input  ParamDataTypeStr=Inherit: Same as input
  phase_hat : Outport
  omega_hat : Outport  Port=2
  wires:
  kp3/1 -> omega_hat/1
  Selector/1 -> kp3/1
  bounder2/1(y) -> Sum/1, phase_hat/1  "theta_hat_bounded"
  bounder1/1(y) -> Gain/1  "e_bounded"
  theta/1 -> Sum/2  "theta"
  Unit Delay/1 -> Gain2/1, Gain1/1, Selector/1
  Sum/1 -> bounder1/1(u)  "e"
  Sum1/1 -> Unit Delay/1
  Gain1/1 -> Sum1/2
  Gain2/1 -> bounder2/1(u)  "theta_hat"
  Gain/1 -> Sum1/1

== system sst_cllc_ttype_inv/single_phase_inverter_modB/single phase inverter control/single_phase_inverter_ctrl/single_phase_pll/pi-ctrl ==
  x : Inport
  xref : Inport  Port=2
  1/Ti : Gain  Gain=kp  SaturateOnIntegerOverflow=on  OutDataTypeStr=Inherit: Same as input  ParamDataTypeStr=Inherit: Same as input
  Saturation : Saturate  UpperLimit=sat_pos  LowerLimit=sat_neg
  Sum1 : Sum  Inputs=+++  SaturateOnIntegerOverflow=on
  Sum2 : Sum  Inputs=-+  SaturateOnIntegerOverflow=on
  Sum3 : Sum  Inputs=-+  SaturateOnIntegerOverflow=on
  Unit Delay4 : UnitDelay  SampleTime=-1
  kp : Gain  Gain=ki*ts  SaturateOnIntegerOverflow=on  OutDataTypeStr=Inherit: Same as input  ParamDataTypeStr=Inherit: Same as input
  u : Outport
  wires:
  xref/1 -> Sum2/2
  x/1 -> Sum2/1
  kp/1 -> Sum1/2
  Sum2/1 -> kp/1, 1/Ti/1
  1/Ti/1 -> Sum1/1, Sum3/1
  Sum3/1 -> Unit Delay4/1
  Sum1/1 -> Saturation/1
  Unit Delay4/1 -> Sum1/3
  Saturation/1 -> u/1, Sum3/2

== system sst_cllc_ttype_inv/dcdc_cllc_modA/input_current_control/input_current_control/inner_ctrl/current_control/i_ctrl ==
  i_tilde : Inport
  -1 < x < 1 : Saturate  UpperLimit=1  LowerLimit=-1  OutDataTypeStr=double
  1/Ti : Gain  Gain=cllc_ctrl.kp_idc  ParamDataTypeStr=double  OutDataTypeStr=double  SaturateOnIntegerOverflow=on
  Sum1 : Sum  Inputs=+++  SaturateOnIntegerOverflow=on
  Sum4 : Sum  Inputs=-+  SaturateOnIntegerOverflow=on
  Unit Delay4 : UnitDelay  SampleTime=-1
  kp2 : Gain  Gain=cllc_ctrl.ki_idc*glb_time.ts_cllc  ParamDataTypeStr=double  OutDataTypeStr=double  SaturateOnIntegerOverflow=on
  phase_shift : Outport
  wires:
  i_tilde/1 -> kp2/1, 1/Ti/1
  Sum1/1 -> -1 < x < 1/1
  kp2/1 -> Sum1/2
  1/Ti/1 -> Sum1/1, Sum4/1
  Sum4/1 -> Unit Delay4/1
  Unit Delay4/1 -> Sum1/3
  -1 < x < 1/1 -> Sum4/2, phase_shift/1  "phase_shift"

== system sst_cllc_ttype_inv/dcdc_cllc_modA/input_current_control/input_current_control/outer_ctrl/current_control/iout_ctrl ==
  i_tilde : Inport
  -1 < x < 1 : Saturate  UpperLimit=1  LowerLimit=-1  OutDataTypeStr=double
  1/Ti : Gain  Gain=cllc_ctrl.kp_udc  ParamDataTypeStr=double  OutDataTypeStr=double  SaturateOnIntegerOverflow=on
  Sum1 : Sum  Inputs=+++  SaturateOnIntegerOverflow=on
  Sum4 : Sum  Inputs=-+  SaturateOnIntegerOverflow=on
  Unit Delay4 : UnitDelay  SampleTime=-1
  kp2 : Gain  Gain=cllc_ctrl.ki_udc*glb_time.ts_cllc  ParamDataTypeStr=double  OutDataTypeStr=double  SaturateOnIntegerOverflow=on
  phase_shift : Outport
  wires:
  -1 < x < 1/1 -> phase_shift/1, Sum4/2  "phase_shift"
  Unit Delay4/1 -> Sum1/3
  Sum4/1 -> Unit Delay4/1
  1/Ti/1 -> Sum4/1, Sum1/1
  kp2/1 -> Sum1/2
  Sum1/1 -> -1 < x < 1/1
  i_tilde/1 -> 1/Ti/1, kp2/1

== system sst_cllc_ttype_inv/dcdc_cllc_modB/input_current_control/input_current_control/inner_ctrl/current_control/i_ctrl ==
  i_tilde : Inport
  -1 < x < 1 : Saturate  UpperLimit=1  LowerLimit=-1  OutDataTypeStr=double
  1/Ti : Gain  Gain=cllc_ctrl.kp_idc  ParamDataTypeStr=double  OutDataTypeStr=double  SaturateOnIntegerOverflow=on
  Sum1 : Sum  Inputs=+++  SaturateOnIntegerOverflow=on
  Sum4 : Sum  Inputs=-+  SaturateOnIntegerOverflow=on
  Unit Delay4 : UnitDelay  SampleTime=-1
  kp2 : Gain  Gain=cllc_ctrl.ki_idc*glb_time.ts_cllc  ParamDataTypeStr=double  OutDataTypeStr=double  SaturateOnIntegerOverflow=on
  phase_shift : Outport
  wires:
  -1 < x < 1/1 -> phase_shift/1, Sum4/2  "phase_shift"
  Unit Delay4/1 -> Sum1/3
  Sum4/1 -> Unit Delay4/1
  1/Ti/1 -> Sum4/1, Sum1/1
  kp2/1 -> Sum1/2
  Sum1/1 -> -1 < x < 1/1
  i_tilde/1 -> 1/Ti/1, kp2/1

== system sst_cllc_ttype_inv/dcdc_cllc_modB/input_current_control/input_current_control/outer_ctrl/current_control/iout_ctrl ==
  i_tilde : Inport
  -1 < x < 1 : Saturate  UpperLimit=1  LowerLimit=-1  OutDataTypeStr=double
  1/Ti : Gain  Gain=cllc_ctrl.kp_udc  ParamDataTypeStr=double  OutDataTypeStr=double  SaturateOnIntegerOverflow=on
  Sum1 : Sum  Inputs=+++  SaturateOnIntegerOverflow=on
  Sum4 : Sum  Inputs=-+  SaturateOnIntegerOverflow=on
  Unit Delay4 : UnitDelay  SampleTime=-1
  kp2 : Gain  Gain=cllc_ctrl.ki_udc*glb_time.ts_cllc  ParamDataTypeStr=double  OutDataTypeStr=double  SaturateOnIntegerOverflow=on
  phase_shift : Outport
  wires:
  i_tilde/1 -> kp2/1, 1/Ti/1
  Sum1/1 -> -1 < x < 1/1
  kp2/1 -> Sum1/2
  1/Ti/1 -> Sum1/1, Sum4/1
  Sum4/1 -> Unit Delay4/1
  Unit Delay4/1 -> Sum1/3
  -1 < x < 1/1 -> Sum4/2, phase_shift/1  "phase_shift"

== system sst_cllc_ttype_inv/single_phase_inverter_modA/single phase inverter control/single_phase_inverter_ctrl/single_phase_current_control/dqpi_current_controller/alphabeta2dq ==
  alpha : Inport
  beta : Inport  Port=2
  MATLAB Function : MATLAB Function  TreatAsAtomicUnit=on
  "d " : Outport  VectorParamsAs1DForOutWhenUnconnected=off
  "q " : Outport  Port=2  VectorParamsAs1DForOutWhenUnconnected=off
  wires:
  alpha/1 -> MATLAB Function/1(alpha)
  beta/1 -> MATLAB Function/2(beta)
  MATLAB Function/1(d) -> "d "/1
  MATLAB Function/2(q) -> "q "/1
  [phase_grid] -> MATLAB Function/3(phase)

== system sst_cllc_ttype_inv/single_phase_inverter_modA/single phase inverter control/single_phase_inverter_ctrl/single_phase_current_control/dqpi_current_controller/dq2alphabeta ==
  d : Inport
  q : Inport  Port=2
  MATLAB Function : MATLAB Function  TreatAsAtomicUnit=on
  alpha : Outport  VectorParamsAs1DForOutWhenUnconnected=off
  wires:
  d/1 -> MATLAB Function/1(d)
  q/1 -> MATLAB Function/2(q)
  MATLAB Function/1(alpha) -> alpha/1
  [phase_grid] -> MATLAB Function/3(phase)

== system sst_cllc_ttype_inv/single_phase_inverter_modA/single phase inverter control/single_phase_inverter_ctrl/single_phase_current_control/dqpi_current_controller/dq_vector_pi ==
  id_ref : Inport
  id : Inport  Port=2
  iq : Inport  Port=3
  iq_ref : Inport  Port=4
  dq_vector_pi : dq_vector_pi/dq_vector_pi  kp=single_phase_inverter_ctrl.kp_inv  ki=single_phase_inverter_ctrl.ki_inv  ts=glb_time.ts_inv  lim_ctrl_out=single_phase_inverter_ctrl.u_lim  CTRPIFF_CLIP_RELEASE=CTRPIFF_CLIP_RELEASE
  ud_ctrl : Outport
  uq_ctrl : Outport  Port=2
  wires:
  id_ref/1 -> dq_vector_pi/1  "id_ref"
  iq_ref/1 -> dq_vector_pi/3  "iq_ref"
  dq_vector_pi/1 -> ud_ctrl/1  "ud_ctrl"
  iq/1 -> dq_vector_pi/4  "iq"
  id/1 -> dq_vector_pi/2  "id"
  dq_vector_pi/2 -> uq_ctrl/1  "uq_ctrl"
  [dclink_voltage_pu] -> dq_vector_pi/5

== system sst_cllc_ttype_inv/single_phase_inverter_modA/single phase inverter control/single_phase_inverter_ctrl/single_phase_current_control/dqpi_current_controller/i2alphabeta ==
  i_alpha : Inport
  FHTalpha : Subsystem
  i_alpha_out : Outport
  i_beta_out : Outport  Port=2
  wires:
  i_alpha/1 -> FHTalpha/1(u)
  FHTalpha/1(ualpha) -> i_alpha_out/1  "u_fht_alpha"
  FHTalpha/2(ubeta) -> i_beta_out/1  "v_fht_alpha"

== system sst_cllc_ttype_inv/single_phase_inverter_modB/single phase inverter control/single_phase_inverter_ctrl/single_phase_current_control/dqpi_current_controller/alphabeta2dq ==
  alpha : Inport
  beta : Inport  Port=2
  MATLAB Function : MATLAB Function  TreatAsAtomicUnit=on
  "d " : Outport  VectorParamsAs1DForOutWhenUnconnected=off
  "q " : Outport  Port=2  VectorParamsAs1DForOutWhenUnconnected=off
  wires:
  [phase_grid] -> MATLAB Function/3(phase)
  MATLAB Function/2(q) -> "q "/1
  MATLAB Function/1(d) -> "d "/1
  beta/1 -> MATLAB Function/2(beta)
  alpha/1 -> MATLAB Function/1(alpha)

== system sst_cllc_ttype_inv/single_phase_inverter_modB/single phase inverter control/single_phase_inverter_ctrl/single_phase_current_control/dqpi_current_controller/dq2alphabeta ==
  d : Inport
  q : Inport  Port=2
  MATLAB Function : MATLAB Function  TreatAsAtomicUnit=on
  alpha : Outport  VectorParamsAs1DForOutWhenUnconnected=off
  wires:
  [phase_grid] -> MATLAB Function/3(phase)
  MATLAB Function/1(alpha) -> alpha/1
  q/1 -> MATLAB Function/2(q)
  d/1 -> MATLAB Function/1(d)

== system sst_cllc_ttype_inv/single_phase_inverter_modB/single phase inverter control/single_phase_inverter_ctrl/single_phase_current_control/dqpi_current_controller/dq_vector_pi ==
  id_ref : Inport
  id : Inport  Port=2
  iq : Inport  Port=3
  iq_ref : Inport  Port=4
  dq_vector_pi : dq_vector_pi/dq_vector_pi  kp=single_phase_inverter_ctrl.kp_inv  ki=single_phase_inverter_ctrl.ki_inv  ts=glb_time.ts_inv  lim_ctrl_out=single_phase_inverter_ctrl.u_lim  CTRPIFF_CLIP_RELEASE=CTRPIFF_CLIP_RELEASE
  ud_ctrl : Outport
  uq_ctrl : Outport  Port=2
  wires:
  [dclink_voltage_pu] -> dq_vector_pi/5
  dq_vector_pi/2 -> uq_ctrl/1  "uq_ctrl"
  id/1 -> dq_vector_pi/2  "id"
  iq/1 -> dq_vector_pi/4  "iq"
  dq_vector_pi/1 -> ud_ctrl/1  "ud_ctrl"
  iq_ref/1 -> dq_vector_pi/3  "iq_ref"
  id_ref/1 -> dq_vector_pi/1  "id_ref"

== system sst_cllc_ttype_inv/single_phase_inverter_modB/single phase inverter control/single_phase_inverter_ctrl/single_phase_current_control/dqpi_current_controller/i2alphabeta ==
  i_alpha : Inport
  FHTalpha : Subsystem
  i_alpha_out : Outport
  i_beta_out : Outport  Port=2
  wires:
  FHTalpha/2(ubeta) -> i_beta_out/1  "v_fht_alpha"
  FHTalpha/1(ualpha) -> i_alpha_out/1  "u_fht_alpha"
  i_alpha/1 -> FHTalpha/1(u)

== system sst_cllc_ttype_inv/single_phase_inverter_modA/single phase inverter control/single_phase_inverter_ctrl/single_phase_current_control/dqpi_current_controller/i2alphabeta/FHTalpha ==
  u : Inport
  Gain : Gain  Gain=single_phase_inverter_ctrl.fht_load.Ld_fht  Multiplication=Matrix(K*u)
  Gain1 : Gain  Gain=single_phase_inverter_ctrl.fht_load.Ad_fht  Multiplication=Matrix(K*u)
  Gain2 : Gain  Gain=single_phase_inverter_ctrl.fht_load.Cfht  Multiplication=Matrix(K*u)
  Gain3 : Gain  Gain=-1/single_phase_inverter_ctrl.omega_base
  Selector : Selector  InputPortWidth=2  IndexOptions=Index vector (dialog)  Indices=1  OutputSizes=1
  Selector1 : Selector  InputPortWidth=2  IndexOptions=Index vector (dialog)  Indices=2  OutputSizes=1
  Sum : Sum  Inputs=-+|
  Sum1 : Sum  Inputs=|++
  Unit Delay : UnitDelay  SampleTime=-1
  ualpha : Outport
  ubeta : Outport  Port=2
  wires:
  u/1 -> Sum/2
  Unit Delay/1 -> Gain2/1, Selector1/1, Selector/1, Gain1/1
  Sum/1 -> Gain/1
  Sum1/1 -> Unit Delay/1
  Gain1/1 -> Sum1/2
  Gain2/1 -> Sum/1
  Selector/1 -> ualpha/1
  Gain/1 -> Sum1/1
  Selector1/1 -> Gain3/1
  Gain3/1 -> ubeta/1

== system sst_cllc_ttype_inv/single_phase_inverter_modB/single phase inverter control/single_phase_inverter_ctrl/single_phase_current_control/dqpi_current_controller/i2alphabeta/FHTalpha ==
  u : Inport
  Gain : Gain  Gain=single_phase_inverter_ctrl.fht_load.Ld_fht  Multiplication=Matrix(K*u)
  Gain1 : Gain  Gain=single_phase_inverter_ctrl.fht_load.Ad_fht  Multiplication=Matrix(K*u)
  Gain2 : Gain  Gain=single_phase_inverter_ctrl.fht_load.Cfht  Multiplication=Matrix(K*u)
  Gain3 : Gain  Gain=-1/single_phase_inverter_ctrl.omega_base
  Selector : Selector  InputPortWidth=2  IndexOptions=Index vector (dialog)  Indices=1  OutputSizes=1
  Selector1 : Selector  InputPortWidth=2  IndexOptions=Index vector (dialog)  Indices=2  OutputSizes=1
  Sum : Sum  Inputs=-+|
  Sum1 : Sum  Inputs=|++
  Unit Delay : UnitDelay  SampleTime=-1
  ualpha : Outport
  ubeta : Outport  Port=2
  wires:
  Gain3/1 -> ubeta/1
  Selector1/1 -> Gain3/1
  Gain/1 -> Sum1/1
  Selector/1 -> ualpha/1
  Gain2/1 -> Sum/1
  Gain1/1 -> Sum1/2
  Sum1/1 -> Unit Delay/1
  Sum/1 -> Gain/1
  Unit Delay/1 -> Gain1/1, Selector/1, Selector1/1, Gain2/1
  u/1 -> Sum/2

== matlab function sst_cllc_ttype_inv/single_phase_inverter_modB/single phase inverter control/single_phase_inverter_ctrl/single_phase_pll/alphabeta2xieta ==
  data: alpha input; xi output; beta input; gamma input; eta output
function [xi,eta] = alphabeta2xieta(alpha,beta,gamma)
    xi  =  alpha*cos(gamma) + beta*sin(gamma);
    eta = -alpha*sin(gamma) + beta*cos(gamma);
end

== matlab function sst_cllc_ttype_inv/single_phase_inverter_modB/single phase inverter control/single_phase_inverter_ctrl/single_phase_pll/bounder2 ==
  data: u input; y output
function y = bounder(u)
    
    y = -pi + mod(u+3*pi,2*pi);
   
end

== matlab function sst_cllc_ttype_inv/single_phase_inverter_modB/single phase inverter control/single_phase_inverter_ctrl/single_phase_pll/double_integrator_observer/bounder1 ==
  data: u input; y output
function y = bounder(u)
    
    y = -pi + mod(u+3*pi,2*pi);
   
end

== matlab function sst_cllc_ttype_inv/single_phase_inverter_modB/single phase inverter control/single_phase_inverter_ctrl/single_phase_pll/double_integrator_observer/bounder2 ==
  data: u input; y output
function y = bounder(u)
    
    y = -pi + mod(u+3*pi,2*pi);
   
end

== matlab function sst_cllc_ttype_inv/single_phase_inverter_modB/single phase inverter control/single_phase_inverter_ctrl/single_phase_pll/xieta2alphabeta ==
  data: xi input; alpha output; eta input; gamma input; beta output
function [alpha,beta] = xieta2alphabeta(xi,eta,gamma)
    alpha  = xi*cos(gamma) - eta*sin(gamma);
    beta = xi*sin(gamma) + eta*cos(gamma);
end

== matlab function sst_cllc_ttype_inv/single_phase_inverter_modA/single phase inverter control/single_phase_inverter_ctrl/single_phase_pll/double_integrator_observer/bounder1 ==
  data: u input; y output
function y = bounder(u)
    
    y = -pi + mod(u+3*pi,2*pi);
   
end

== matlab function sst_cllc_ttype_inv/single_phase_inverter_modA/single phase inverter control/single_phase_inverter_ctrl/single_phase_pll/double_integrator_observer/bounder2 ==
  data: u input; y output
function y = bounder(u)
    
    y = -pi + mod(u+3*pi,2*pi);
   
end

== matlab function sst_cllc_ttype_inv/single_phase_inverter_modA/single phase inverter control/single_phase_inverter_ctrl/single_phase_pll/xieta2alphabeta ==
  data: xi input; alpha output; eta input; gamma input; beta output
function [alpha,beta] = xieta2alphabeta(xi,eta,gamma)
    alpha  = xi*cos(gamma) - eta*sin(gamma);
    beta = xi*sin(gamma) + eta*cos(gamma);
end

== matlab function sst_cllc_ttype_inv/line_source/phase_gen/bounder1 ==
  data: u input; y output
function y = bounder(u)
    
    y = -pi + mod(u+3*pi,2*pi);
end
